simulink model "GUI_LAST"  (Simulink 8.0)
settings: Solver=ode45  StartTime=0.0  StopTime=inf  FixedStep=Ts  RelTol=1e-3
InitFcn:
  | Ts = 0.001;
  | temp1 = 0;
  | temp2 = 0;
  | temp3 = 0;
  | temp4 = 0;
  | voltage_cap1 = 0;
  | voltage_cap2 = 0;
undefined symbols (not defined in the file or in its folder): serial
libraries: instrumentlib x3
settings Model: Creator=julien  LastModifiedBy=julien

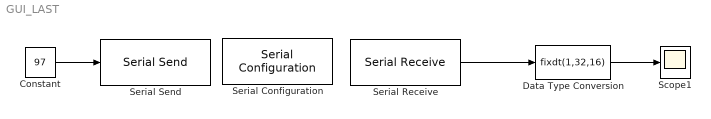
== system GUI_LAST ==
  Constant : Constant  Value=97  OutDataTypeStr=uint8  SampleTime=Ts
  Data Type Conversion : DataTypeConversion  OutDataTypeStr=fixdt(1,32,16)  ConvertRealWorld=Stored Integer (SI)  SampleTime=Ts  LockScale=on
  Scope1 : Scope
      settings: TimeRange=0.1  YMin=0  YMax=0.065  SampleInput=on  SampleTime=Ts
  Serial Configuration : instrumentlib/Serial Configuration  Priority=-200000  ComPortMenu=COM4  ComPort=COM4  ObjConstructor=serial('COM4');  BaudRate=520834  DataBits=8  Parity=none  StopBits=1  FlowControl=none  Timeout=10  ByteOrder=LittleEndian
  Serial Receive : instrumentlib/Serial Receive  ComPortMenu=COM4  ComPort=COM4  ObjConstructor=serial('COM4');  Terminator=<none>  DataSize=[1 1]  DataType=uint32  EnableBlockingMode=on  ActionDataUnavailable=Output last received value  CustomValue=0  SampleTime=0.001
  Serial Send : instrumentlib/Serial Send  ComPortMenu=COM4  ComPort=COM4  ObjConstructor=serial('COM4');  Terminator=<none>  EnableBlockingMode=on
  wires:
  Serial Receive/1 -> Data Type Conversion/1
  Data Type Conversion/1 -> Scope1/1
  Constant/1 -> Serial Send/1
